simulink model "CL2MGR"  (R2024a)
settings: Solver=VariableStepAuto  StartTime=0.0  StopTime=10.0  RelTol=1e-3
settings Model: Creator=jeonghyun  LastModifiedBy=gluts

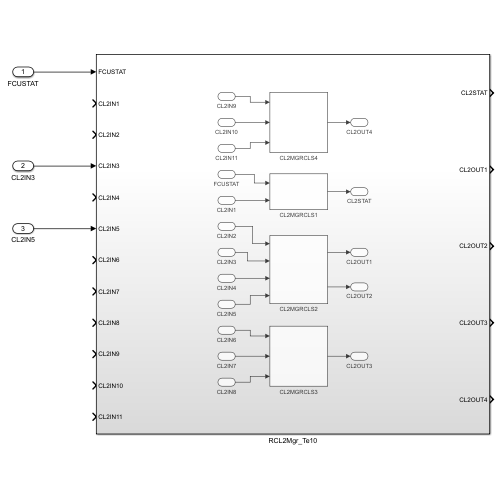
[thumbnail: Simulink's stored preview of the top-level diagram]
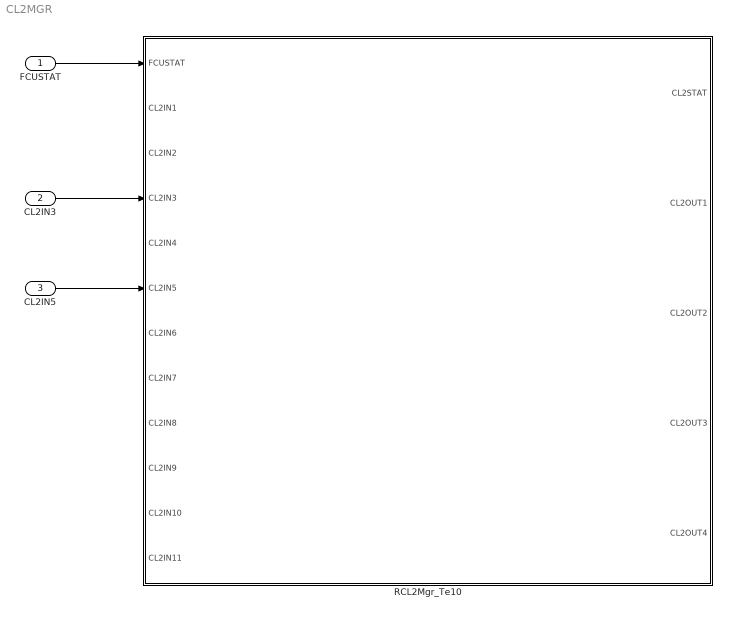
== system CL2MGR ==
  FCUSTAT : Inport
  CL2IN3 : Inport  Port=2
  CL2IN5 : Inport  Port=3
  RCL2Mgr_Te10 : Subsystem
  wires:
  CL2IN3/1 -> RCL2Mgr_Te10/4(CL2IN3)
  FCUSTAT/1 -> RCL2Mgr_Te10/1(FCUSTAT)
  CL2IN5/1 -> RCL2Mgr_Te10/6(CL2IN5)

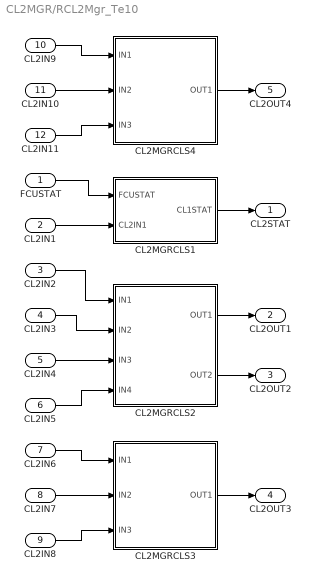
== system CL2MGR/RCL2Mgr_Te10 ==
  FCUSTAT : Inport
  CL2IN1 : Inport  Port=2
  CL2IN2 : Inport  Port=3
  CL2IN3 : Inport  Port=4
  CL2IN4 : Inport  Port=5
  CL2IN5 : Inport  Port=6
  CL2IN6 : Inport  Port=7
  CL2IN7 : Inport  Port=8
  CL2IN8 : Inport  Port=9
  CL2IN9 : Inport  Port=10
  CL2IN10 : Inport  Port=11
  CL2IN11 : Inport  Port=12
  CL2MGRCLS1 : Subsystem
  CL2MGRCLS2 : Subsystem
  CL2MGRCLS3 : Subsystem
  CL2MGRCLS4 : Subsystem
  CL2STAT : Outport
  CL2OUT1 : Outport  Port=2
  CL2OUT2 : Outport  Port=3
  CL2OUT3 : Outport  Port=4
  CL2OUT4 : Outport  Port=5
  wires:
  CL2IN5/1 -> CL2MGRCLS2/4(IN4)
  CL2IN2/1 -> CL2MGRCLS2/1(IN1)
  CL2IN3/1 -> CL2MGRCLS2/2(IN2)
  CL2IN4/1 -> CL2MGRCLS2/3(IN3)
  CL2IN9/1 -> CL2MGRCLS4/1(IN1)
  CL2IN1/1 -> CL2MGRCLS1/2(CL2IN1)
  CL2MGRCLS1/1(CL1STAT) -> CL2STAT/1
  CL2IN10/1 -> CL2MGRCLS4/2(IN2)
  CL2IN11/1 -> CL2MGRCLS4/3(IN3)
  FCUSTAT/1 -> CL2MGRCLS1/1(FCUSTAT)
  CL2IN8/1 -> CL2MGRCLS3/3(IN3)
  CL2IN7/1 -> CL2MGRCLS3/2(IN2)
  CL2IN6/1 -> CL2MGRCLS3/1(IN1)
  CL2MGRCLS4/1(OUT1) -> CL2OUT4/1
  CL2MGRCLS2/1(OUT1) -> CL2OUT1/1
  CL2MGRCLS2/2(OUT2) -> CL2OUT2/1
  CL2MGRCLS3/1(OUT1) -> CL2OUT3/1

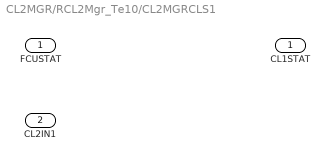
== system CL2MGR/RCL2Mgr_Te10/CL2MGRCLS1 ==
  FCUSTAT : Inport
  CL2IN1 : Inport  Port=2
  CL1STAT : Outport

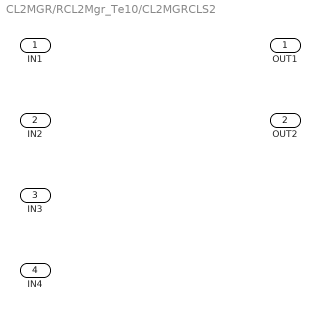
== system CL2MGR/RCL2Mgr_Te10/CL2MGRCLS2 ==
  IN1 : Inport
  IN2 : Inport  Port=2
  IN3 : Inport  Port=3
  IN4 : Inport  Port=4
  OUT1 : Outport
  OUT2 : Outport  Port=2

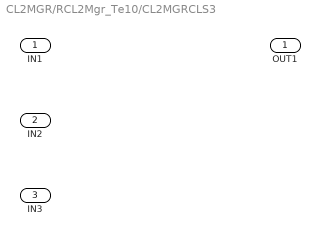
== system CL2MGR/RCL2Mgr_Te10/CL2MGRCLS3 ==
  IN1 : Inport
  IN2 : Inport  Port=2
  IN3 : Inport  Port=3
  OUT1 : Outport

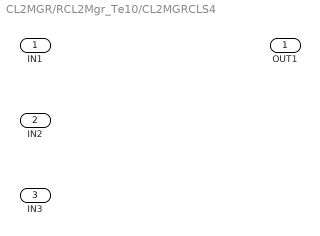
== system CL2MGR/RCL2Mgr_Te10/CL2MGRCLS4 ==
  IN1 : Inport
  IN2 : Inport  Port=2
  IN3 : Inport  Port=3
  OUT1 : Outport
